simulink model "Fuzzy_PID_1"  (Simulink 8.4)
settings: Solver=ode45  StartTime=0.0  StopTime=10.0  RelTol=1e-3
undefined symbols (not defined in the file or in its folder): sigbuilder_block
libraries: fuzblock x1, simulink x1
settings Model: Creator=Administrator  LastModifiedBy=Administrator

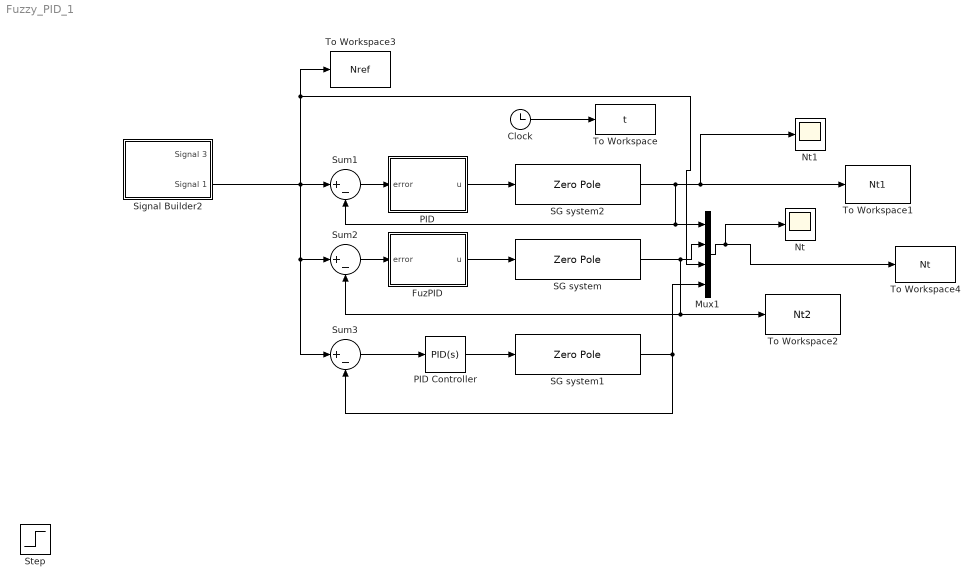
== system Fuzzy_PID_1 ==
  Clock : Clock
  FuzPID : Subsystem  mask{Kp=2.5, Ki=1.4, Kd=0, dKp=0.4, dKi=0.2, dKd=0, Ke=0, Kec=0.1}
      mask prompts: Kp "Proportional(Kp)"; Ki "Integral(Ki)"; Kd "Derivative(Kd)"; dKp "DeltaProportional(dKp)"; dKi "DeltaIntegral(dKi)"; dKd "DeltaDerivative(dKd)"; Ke "factor of error"; Kec "factor of de/dt"
      mask Display: disp('Fuzzy PID')
  Mux1 : Mux
  Nt : Scope
      settings: TimeRange=0.5  YMin=0.45  YMax=1.15
  Nt1 : Scope
      settings: TimeRange=0.5  YMin=0.955  YMax=1.025
  PID : Subsystem  mask{Kp=2.5, Ki=1.4, Kd=0}
      mask prompts: Kp "Proportional(Kp)"; Ki "Integral(Ki)"; Kd "Derivative(Kd)"
      mask help: Traditonal PID controller with three parameters:Proportional(Kp),Integral(Ki) and Derivative(Kd)
      mask Display: disp('PID Controller')
  PID Controller : simulink/Continuous/PID Controller  Controller=PID  TimeDomain=Continuous-time  SampleTime=-1  IntegratorMethod=Forward Euler  FilterMethod=Forward Euler  Form=Parallel  P=0.999855740158371  I=3.45901912667025  D=0  N=100  InitialConditionSource=internal  InitialConditionForIntegrator=0  InitialConditionForFilter=0  ExternalReset=none  LimitOutput=off  UpperSaturationLimit=inf  LowerSaturationLimit=-inf  LinearizeAsGain=on  AntiWindupMode=none  Kb=1  TrackingMode=off  Kt=1  PParamMin=[]  PParamMax=[]  IParamMin=[]  IParamMax=[]  DParamMin=[]  DParamMax=[]  NParamMin=[]  NParamMax=[]  KbParamMin=[]  KbParamMax=[]  KtParamMin=[]  KtParamMax=[]  POutMin=[]  POutMax=[]  IOutMin=[]  IOutMax=[]  DOutMin=[]  DOutMax=[]  NOutMin=[]  NOutMax=[]  KbOutMin=[]  KbOutMax=[]  KtOutMin=[]  KtOutMax=[]  IntegratorOutMin=[]  IntegratorOutMax=[]  FilterOutMin=[]  FilterOutMax=[]  SumOutMin=[]  SumOutMax=[]  SumI1OutMin=[]  SumI1OutMax=[]  SumI2OutMin=[]  SumI2OutMax=[]  SumI3OutMin=[]  SumI3OutMax=[]  SumDOutMin=[]  SumDOutMax=[]  SaturationOutMin=[]  SaturationOutMax=[]  IntegratorContinuousStateAttributes=''  IntegratorStateMustResolveToSignalObject=off  IntegratorRTWStateStorageClass=Auto  FilterContinuousStateAttributes=''  FilterStateMustResolveToSignalObject=off  FilterRTWStateStorageClass=Auto  DifferentiatorICPrevScaledInput=0  DifferentiatorOutMin=[]  DifferentiatorOutMax=[]  UseFilter=on
  SG system : ZeroPole  Zeros=[]  Poles=[-2.865 -40.235 ]  Gain=792
  SG system1 : ZeroPole  Zeros=[]  Poles=[-2.865 -40.235]  Gain=792
  SG system2 : ZeroPole  Zeros=[]  Poles=[-2.865 -40.235]  Gain=792
  Signal Builder2 : Subsystem  Tag=STV Subsys  LoadFcn=sigbuilder_block('load');  StartFcn=sigbuilder_block('start');  StopFcn=sigbuilder_block('stop');  ClipboardFcn=sigbuilder_block('clipboard');  mask(Sigbuilder block){}
      mask help: Sigbuilder GUI
      mask init:
      | if ~strcmp(get_param(bdroot(gcbh),'SimulationStatus'),'stopped') tuvar = sigbuilder_block('maskInit'); end
      settings: CopyFcn=sigbuilder_block('copy');  DeleteFcn=sigbuilder_block('delete');  ModelCloseFcn=sigbuilder_block('modelClose');  PreSaveFcn=sigbuilder_block('preSave');  PauseFcn=sigbuilder_block('pause')  ContinueFcn=sigbuilder_block('continue')  NameChangeFcn=sigbuilder_block('namechange');  OpenFcn=sigbuilder_block('open',[-15.75 97.5 954 496.5 ]);  CloseFcn=sigbuilder_block('close');
      mask Display: plot(0,0,100,100,[10,10,40,40,10],[80,20,20,80,80],[40,10],[50,50], [40,27,10],[65,72,56],[40,25,25,10],[28,28,43,43]);
  Step : Step  Time=0  SampleTime=0
  Sum1 : Sum  Inputs=|+-
  Sum2 : Sum  Inputs=|+-
  Sum3 : Sum  Inputs=|+-
  To Workspace : ToWorkspace  VariableName=t  SampleTime=0.0001
  To Workspace1 : ToWorkspace  VariableName=Nt1  SampleTime=0.0001
  To Workspace2 : ToWorkspace  VariableName=Nt2  SampleTime=0.0001
  To Workspace3 : ToWorkspace  VariableName=Nref  SampleTime=0.0001
  To Workspace4 : ToWorkspace  VariableName=Nt  SampleTime=0.0001
  wires:
  PID/1(u) -> SG system2/1
  Sum1/1 -> PID/1(error)
  Mux1/1 -> To Workspace4/1, Nt/1
  FuzPID/1(u) -> SG system/1
  SG system/1 -> Sum2/2, To Workspace2/1, Mux1/2
  Sum2/1 -> FuzPID/1(error)
  SG system2/1 -> Sum1/2, Mux1/1, To Workspace1/1, Nt1/1
  Clock/1 -> To Workspace/1
  PID Controller/1 -> SG system1/1
  Sum3/1 -> PID Controller/1
  SG system1/1 -> Sum3/2, Mux1/4
  Signal Builder2/2(Signal 1) -> Mux1/3, To Workspace3/1, Sum3/1, Sum2/1, Sum1/1

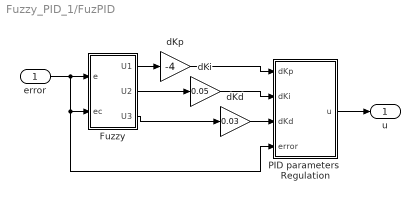
== system Fuzzy_PID_1/FuzPID ==
  error : Inport
  Fuzzy : Subsystem  mask{Ke=Ke, Kec=Kec}
      mask prompts: Ke "factor of error"; Kec "factor of de/dt"
      mask help: Fuzzy Bolck
      mask Display: disp('Fuzzy')
  PID parameters  Regulation : Subsystem  mask{Kp=Kp, Ki=Ki, Kd=Kd}
      mask prompts: Kp "Proportional(Kp)"; Ki "Integral(Ki)"; Kd "Derivative(Kd)"
      mask Display: disp('PID\nRegulation')
  dKd : Gain  Gain=0.03
  dKi : Gain  Gain=0.05
  dKp : Gain  Gain=-4
  u : Outport
  wires:
  error/1 -> Fuzzy/1(e), Fuzzy/2(ec), PID parameters  Regulation/4(error)
  Fuzzy/1(U1) -> dKp/1
  Fuzzy/2(U2) -> dKi/1
  Fuzzy/3(U3) -> dKd/1
  dKp/1 -> PID parameters  Regulation/1(dKp)
  dKi/1 -> PID parameters  Regulation/2(dKi)
  dKd/1 -> PID parameters  Regulation/3(dKd)
  PID parameters  Regulation/1(u) -> u/1

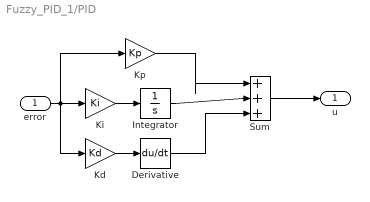
== system Fuzzy_PID_1/PID ==
  error : Inport
  Derivative : Derivative
  Integrator : Integrator
  Kd : Gain  Gain=Kd
  Ki : Gain  Gain=Ki
  Kp : Gain  Gain=Kp
  Sum : Sum  Inputs=|+++
  u : Outport
  wires:
  error/1 -> Kp/1, Ki/1, Kd/1
  Ki/1 -> Integrator/1
  Kd/1 -> Derivative/1
  Kp/1 -> Sum/1
  Integrator/1 -> Sum/2
  Derivative/1 -> Sum/3
  Sum/1 -> u/1

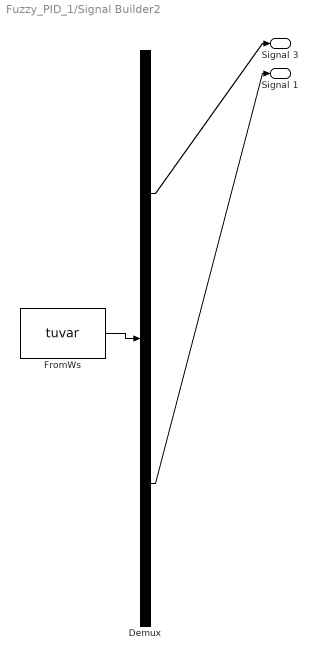
== system Fuzzy_PID_1/Signal Builder2 ==
  Demux : Demux  Tag=STV Demux  Outputs=2
  FromWs : FromWorkspace  Tag=STV FromWs  VariableName=tuvar  SampleTime=0  SigBuilderData=DataTag0  VnvData=DataTag1
      SigBuilderData=|
      | common.afterFinalStr = 'Extrapolate'
      | common.sampleTime = 0
      | dataSet.timeRange = [0 1]
      | dataSet.name = 'Group 1'
      | sbobj.Groups.Name = 'Group 1'
      | sbobj.Groups.Signals(1).Name = 'Signal 3'
      | sbobj.Groups.Signals(1).XData = [0 0.6 0.6 0.610526315789 0.621052631579 0.631578947368 0.642105263158 0.652631578947 0.663157894737 0.673684210526 0.684210526316 0.694736842105 0.705263157895 0.715789473684 0.726315789474 0.736842105263 0.747368421053 0.757894736842 0.768421052632 0.778947368421 0.789473684211 0.8 1]
      | sbobj.Groups.Signals(1).YData = [1 1 1 0.983540540972 0.96753005308 0.952405260696 0.938578728731 0.926427608933 0.916283352174 0.908422667334 0.903059973406 0.900341550699 0.900341550699 0.903059973406 0.908422667334 0.916283352174 0.926427608933 0.938578728731 0.952405260696 0.96753005308 0.983540540972 1 1]
      | sbobj.Groups.Signals(2).Name = 'Signal 1'
      | sbobj.Groups.Signals(2).XData = [0 0.5 0.5 10]
      | sbobj.Groups.Signals(2).YData = [0 0 1 1]
  Signal 3 : Outport  Tag=STV Outport
  Signal 1 : Outport  Tag=STV Outport  Port=2
  wires:
  FromWs/1 -> Demux/1
  Demux/1 -> Signal 3/1
  Demux/2 -> Signal 1/1

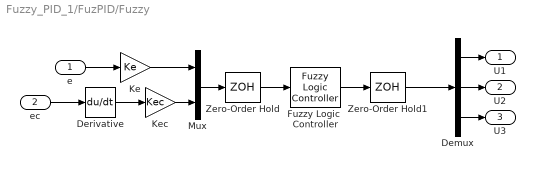
== system Fuzzy_PID_1/FuzPID/Fuzzy ==
  e : Inport
  ec : Inport  Port=2
  Demux : Demux  Outputs=3
  Derivative : Derivative
  Fuzzy Logic  Controller : fuzblock/Fuzzy Logic  Controller  fis=fuzzyPID
  Ke : Gain  Gain=Ke
  Kec : Gain  Gain=Kec
  Mux : Mux  Inputs=2
  Zero-Order Hold : ZeroOrderHold  SampleTime=0.005
  Zero-Order Hold1 : ZeroOrderHold  SampleTime=0.005
  U1 : Outport
  U2 : Outport  Port=2
  U3 : Outport  Port=3
  wires:
  Derivative/1 -> Kec/1
  Zero-Order Hold/1 -> Fuzzy Logic  Controller/1
  Mux/1 -> Zero-Order Hold/1
  Kec/1 -> Mux/2
  Ke/1 -> Mux/1
  Fuzzy Logic  Controller/1 -> Zero-Order Hold1/1
  e/1 -> Ke/1
  ec/1 -> Derivative/1
  Demux/1 -> U1/1
  Demux/2 -> U2/1
  Demux/3 -> U3/1
  Zero-Order Hold1/1 -> Demux/1

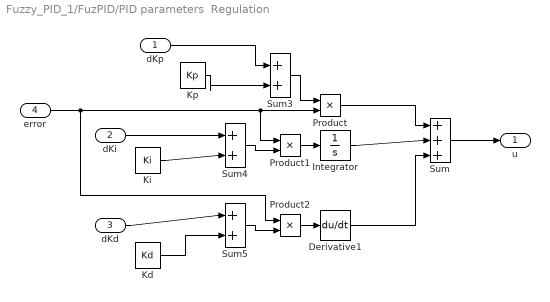
== system Fuzzy_PID_1/FuzPID/PID parameters  Regulation ==
  dKp : Inport
  dKi : Inport  Port=2
  dKd : Inport  Port=3
  error : Inport  Port=4
  Derivative1 : Derivative
  Integrator : Integrator
  Kd : Constant  Value=Kd
  Ki : Constant  Value=Ki
  Kp : Constant  Value=Kp
  Product : Product  RndMeth=Zero
  Product1 : Product  RndMeth=Zero
  Product2 : Product  RndMeth=Zero
  Sum : Sum  Inputs=|+++
  Sum3 : Sum  Inputs=|++
  Sum4 : Sum  Inputs=|++
  Sum5 : Sum  Inputs=|++
  u : Outport
  wires:
  Integrator/1 -> Sum/2
  Derivative1/1 -> Sum/3
  Sum/1 -> u/1
  dKp/1 -> Sum3/1
  Sum3/1 -> Product/1
  error/1 -> Product/2, Product1/1, Product2/1
  Product/1 -> Sum/1
  Kp/1 -> Sum3/2
  dKi/1 -> Sum4/1
  Ki/1 -> Sum4/2
  dKd/1 -> Sum5/1
  Kd/1 -> Sum5/2
  Product1/1 -> Integrator/1
  Sum4/1 -> Product1/2
  Product2/1 -> Derivative1/1
  Sum5/1 -> Product2/2
